simulink model "pll"  (R2024b)
settings: Solver=VariableStepAuto  StartTime=0.0  StopTime=10.0  MaxStep=1e-5  RelTol=1e-3
libraries: slpidlib x1
settings Model: Creator=francesco.bazzani  LastModifiedBy=francesco.bazzani

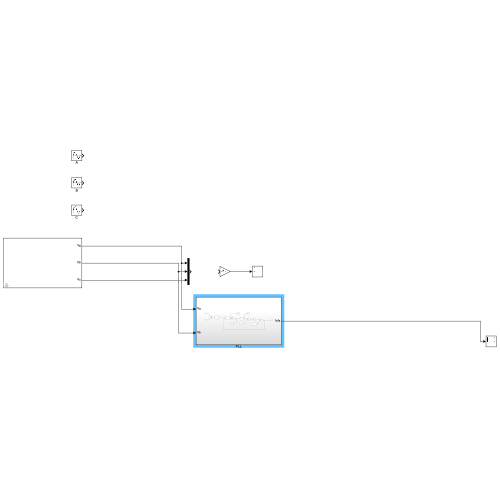
[thumbnail: Simulink's stored preview of the top-level diagram]
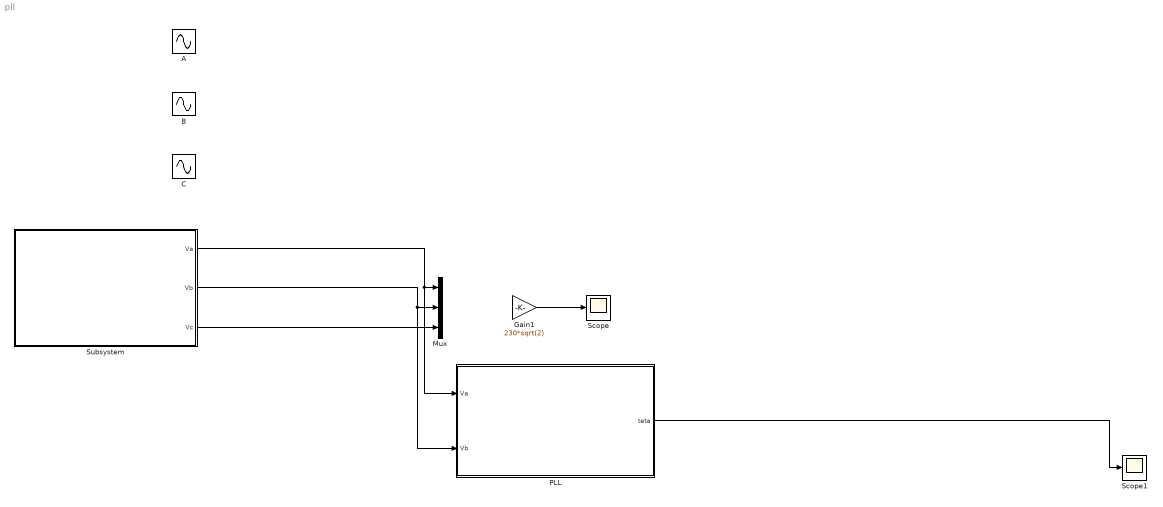
== system pll ==
  A : Sin  Amplitude=230*sqrt(2)  Frequency=2*pi*50  SampleTime=0
  B : Sin  Amplitude=230*sqrt(2)  Frequency=2*pi*50  Phase=2*pi/3  SampleTime=0
  C : Sin  Amplitude=230*sqrt(2)  Frequency=2*pi*50  Phase=-2*pi/3  SampleTime=0
  Gain1 : Gain  Gain=230*sqrt(2)
  Mux : Mux  Inputs=3
  PLL : Subsystem
  Scope : Scope
  Scope1 : Scope
  Subsystem : Subsystem  mask{f=50, Vp=230*sqrt(2)}
      mask prompts: f "Frequency [Hz]"; Vp "Peak value [V]"
  wires:
  Gain1/1 -> Scope/1
  Subsystem/2(Vb) -> PLL/2(Vb), Mux/2
  Subsystem/1(Va) -> PLL/1(Va), Mux/1
  Subsystem/3(Vc) -> Mux/3
  PLL/1(teta) -> Scope1/1

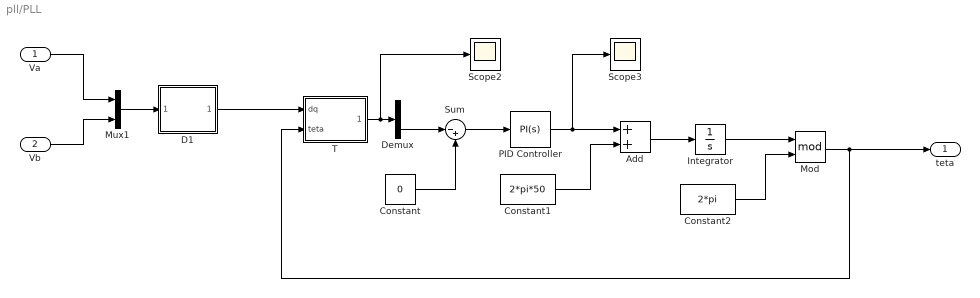
== system pll/PLL ==
  Va : Inport
  Vb : Inport  Port=2
  Add : Sum
  Constant : Constant  Value=0
  Constant1 : Constant  Value=2*pi*50
  Constant2 : Constant  Value=2*pi
  D1 : Subsystem
  Demux : Demux  Outputs=2
  Integrator : Integrator
  Mod : Math  Operator=mod
  Mux1 : Mux  Inputs=2
  PID Controller : slpidlib/PID Controller  Controller=PI  Form=Parallel  TimeDomain=Continuous-time  UseExternalTs=off  SampleTime=-1  IntegratorMethod=Forward Euler  FilterMethod=Forward Euler  ControllerParametersSource=internal  P=2.7  I=1200  UseKiTs=off  D=0  UseExternalDerivativeSource=off  N=100  UseFilter=on  TunerSelectOption=Transfer Function Based (PID Tuner App)  InitialConditionSource=internal  InitialConditionForIntegrator=0  InitialConditionForFilter=0  DifferentiatorICPrevScaledInput=0  ExternalReset=none  TrackingMode=off  Kt=1  LimitOutput=off  SatLimitsSource=internal  UpperSaturationLimit=inf  LowerSaturationLimit=-inf  LinearizeAsGain=on  AntiWindupMode=none  Kb=1  LimitIntegrator=off  UpperIntegratorSaturationLimit=inf  LowerIntegratorSaturationLimit=-inf  POutMin=[]  POutMax=[]  IOutMin=[]  IOutMax=[]  DOutMin=[]  DOutMax=[]  NOutMin=[]  NOutMax=[]  SumOutMin=[]  SumOutMax=[]  SaturationOutMin=[]  SaturationOutMax=[]  PParamMin=[]  PParamMax=[]  IParamMin=[]  IParamMax=[]  DParamMin=[]  DParamMax=[]  NParamMin=[]  NParamMax=[]  KbParamMin=[]  KbParamMax=[]  KtParamMin=[]  KtParamMax=[]  KbOutMin=[]  KbOutMax=[]  KtOutMin=[]  KtOutMax=[]  IntegratorOutMin=[]  IntegratorOutMax=[]  FilterOutMin=[]  FilterOutMax=[]  SumI1OutMin=[]  SumI1OutMax=[]  SumI2OutMin=[]  SumI2OutMax=[]  SumI3OutMin=[]  SumI3OutMax=[]  SumI4OutMin=[]  SumI4OutMax=[]  SumDOutMin=[]  SumDOutMax=[]  DifferentiatorOutMin=[]  DifferentiatorOutMax=[]  FilterDiffOutCoefMin=[]  FilterDiffOutCoefMax=[]  ReciprocalOutMin=[]  ReciprocalOutMax=[]  SumDenOutMin=[]  SumDenOutMax=[]  SumNumOutMin=[]  SumNumOutMax=[]  DivideOutMin=[]  DivideOutMax=[]  UdiffTsProdOutMin=[]  UdiffTsProdOutMax=[]  NTsProdOutMin=[]  NTsProdOutMax=[]  UintegralTsProdOutMin=[]  UintegralTsProdOutMax=[]  UngainTsProdOutMin=[]  UngainTsProdOutMax=[]  ClampingZeroOutDataTypeStr=Inherit: Inherit via back propagation  ClampingZeroOutMin=[]  ClampingZeroOutMax=[]  FilterDenConstantOutDataTypeStr=Inherit: Inherit via back propagation  FilterDenConstantOutMin=[]  FilterDenConstantOutMax=[]  PCopyOutDataTypeStr=Inherit: Inherit via back propagation  PCopyOutMin=[]  PCopyOutMax=[]  NCopyOutDataTypeStr=Inherit: Inherit via back propagation  NCopyOutMin=[]  NCopyOutMax=[]  IntegratorContinuousStateAttributes=''  IntegratorStateMustResolveToSignalObject=off  IntegratorRTWStateStorageClass=Auto  FilterContinuousStateAttributes=''  FilterStateMustResolveToSignalObject=off  FilterRTWStateStorageClass=Auto  ParallelPVariant=InternalParameters  IdealPVariant=Disabled  IVariant=InternalParameters  DVariant=Disabled  IntegratorVariant=Continuous  SatVariant=Disabled  AWVariant=Passthrough  PCopyVariant=Disabled  TRVariant=Disabled  FdbkBlocksVariant=Forward  IdealPFdbkVariant=Disabled  SatFdbkVariant=Disabled  DerivativeFilterVariant=Disabled  NVariant=Disabled  NCopyVariant=Disabled_SignalSpec  FilterICVariant=Disabled  IntegratorICVariant=InternalICs  ExternalResetVariant=Disabled  TRSumVariant=Passthrough  SumFdbkVariant=Disabled  SumVariant=Sum_PI  TsampFilterVariant=InternalTs  TsampNgainVariant=Passthrough  TsampIntegralVariant=Disabled_SignalSpec  ExternalSaturationOutDataTypeStr=Inherit: Same as second input  DerivativeSourceVariant=Disabled  PreIntVariant=InternalPreInt
  Scope2 : Scope
  Scope3 : Scope
  Sum : Sum  Inputs=|-+
  T : Subsystem
  teta : Outport
  wires:
  Vb/1 -> Mux1/2
  Add/1 -> Integrator/1
  Integrator/1 -> Mod/1
  Constant2/1 -> Mod/2
  Constant/1 -> Sum/2
  Va/1 -> Mux1/1
  Constant1/1 -> Add/2
  Sum/1 -> PID Controller/1
  Mux1/1 -> D1/1(ab(c))
  Mod/1 -> teta/1, T/2(teta)
  T/1(dq(teta)) -> Scope2/1, Demux/1
  D1/1(dq(0)) -> T/1(dq)
  PID Controller/1 -> Scope3/1, Add/1
  Demux/2 -> Sum/1

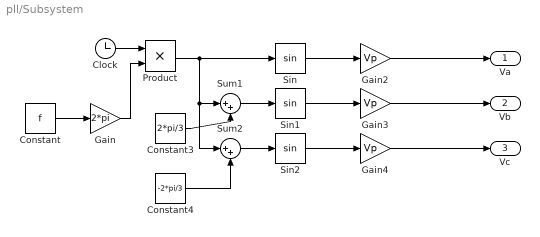
== system pll/Subsystem ==
  Clock : Clock
  Constant : Constant  Value=f
  Constant3 : Constant  Value=2*pi/3
  Constant4 : Constant  Value=-2*pi/3
  Gain : Gain  Gain=2*pi
  Gain2 : Gain  Gain=Vp
  Gain3 : Gain  Gain=Vp
  Gain4 : Gain  Gain=Vp
  Product : Product
  Sin : Trigonometry
  Sin1 : Trigonometry
  Sin2 : Trigonometry
  Sum1 : Sum  Inputs=|++
  Sum2 : Sum  Inputs=|++
  Va : Outport
  Vb : Outport  Port=2
  Vc : Outport  Port=3
  wires:
  Gain4/1 -> Vc/1
  Gain3/1 -> Vb/1
  Sin1/1 -> Gain3/1
  Constant/1 -> Gain/1
  Gain/1 -> Product/2
  Clock/1 -> Product/1
  Sin/1 -> Gain2/1
  Gain2/1 -> Va/1
  Sum1/1 -> Sin1/1
  Sum2/1 -> Sin2/1
  Sin2/1 -> Gain4/1
  Constant3/1 -> Sum1/2
  Constant4/1 -> Sum2/2
  Product/1 -> Sum1/1, Sum2/1, Sin/1

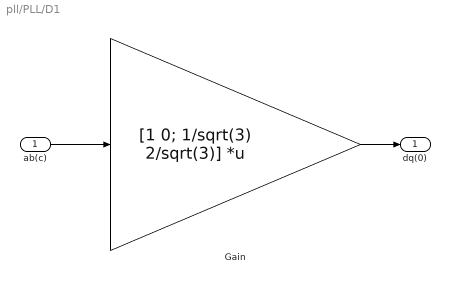
== system pll/PLL/D1 ==
  ab(c) : Inport
  Gain : Gain  Gain=[1 0; 1/sqrt(3) 2/sqrt(3)]  Multiplication=Matrix(K*u)
  dq(0) : Outport
  wires:
  Gain/1 -> dq(0)/1
  ab(c)/1 -> Gain/1

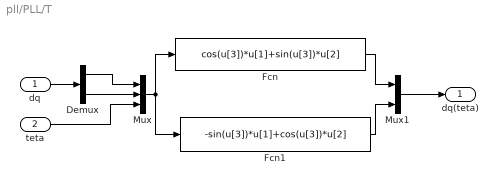
== system pll/PLL/T ==
  dq : Inport
  teta : Inport  Port=2
  Demux : Demux  Outputs=2
  Fcn : Fcn  Expr=cos(u[3])*u[1]+sin(u[3])*u[2]
  Fcn1 : Fcn  Expr=-sin(u[3])*u[1]+cos(u[3])*u[2]
  Mux : Mux  Inputs=3
  Mux1 : Mux  Inputs=2
  dq(teta) : Outport
  wires:
  dq/1 -> Demux/1
  Demux/1 -> Mux/1
  Demux/2 -> Mux/2
  teta/1 -> Mux/3
  Mux/1 -> Fcn1/1, Fcn/1
  Fcn/1 -> Mux1/1
  Fcn1/1 -> Mux1/2
  Mux1/1 -> dq(teta)/1
